simulink model "fp_model"  (R2024a)
settings: Solver=FixedStepAuto  StartTime=0.0  StopTime=10.0  RelTol=1e-3
libraries: dspxfrm3 x1, dspsigops x1
settings Model: Creator=Jan Rosa  LastModifiedBy=Jan Rosa

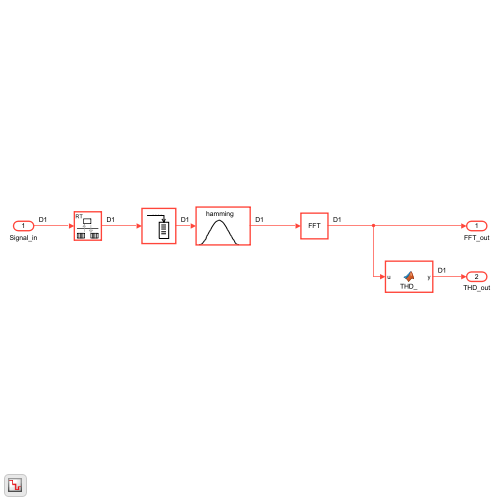
[thumbnail: Simulink's stored preview of the top-level diagram]
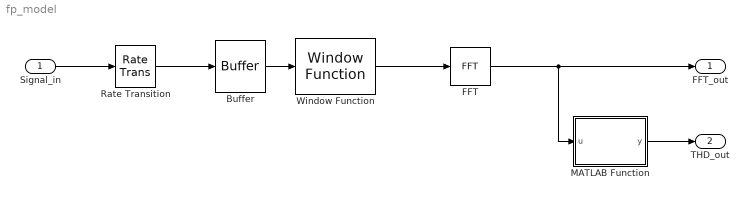
== system fp_model ==
  Signal_in : Inport
  Buffer : Buffer  N=512  V=511  OutputFrames=off
  FFT : dspxfrm3/FFT  FFTImplementation=Auto  CompMethod=Table lookup  TableOpt=NEW  TableOptActive=Speed  BitRevOrder=off  Normalize=off  InheritFFTLength=on  FFTLength=64  WrapInput=on  roundingMode=Ceiling  overflowMode=off  firstCoeffDataTypeStr=Inherit: Same word length as input  firstCoeffLastDataTypeStr=Inherit: Same word length as input  outputMin=[]  outputMax=[]
  MATLAB Function : MATLAB Function  TreatAsAtomicUnit=on
  Rate Transition : RateTransition  OutPortSampleTime=1/29900
  Window Function : dspsigops/Window Function  winmode=Apply window to input  wintype=Hamming  sampmode=Continuous  samptime=1  N=64  Rs=50  beta=10  winsamp=Symmetric  UserWindow=hamming  OptParams=off  UserParams={'symmetric'}  dataType=double  isSigned=on  wordLen=16  udDataType=sfix(16)  fracBitsMode=Best precision  numFracBits=15  roundingMode=Floor  overflowMode=off  numSidelobes=4  sidelobeLevel=-30
  FFT_out : Outport
  THD_out : Outport  Port=2
  wires:
  Window Function/1 -> FFT/1
  FFT/1 -> MATLAB Function/1(u), FFT_out/1
  MATLAB Function/1(y) -> THD_out/1
  Buffer/1 -> Window Function/1
  Signal_in/1 -> Rate Transition/1
  Rate Transition/1 -> Buffer/1

== matlab function fp_model/MATLAB Function ==
  data: u input; y output
function y = THD_(u)

y = abs(u(1)/sum(u));
